simulink model "ex5_potentialFieldsTest_sim"  (R2025b)
settings: Solver=FixedStepAuto  StartTime=0.0  StopTime=15  FixedStep=1/GV.freq  RelTol=1e-3
values from neighbouring files (symbols this model uses):
  Kd = damp*w*2    (= 40)    [ex5_potentialFieldsTest.m]
  Kp = w*w    (= 400)    [ex5_potentialFieldsTest.m]
  vel_lim_max = 2.1750    (= 2.175)    [ex5_potentialFieldsTest.m]
  vel_lim_min = -vel_lim_max    (= -2.175)    [ex5_potentialFieldsTest.m]
libraries: simulink x1
settings Model: Creator=borek  LastModifiedBy=borek

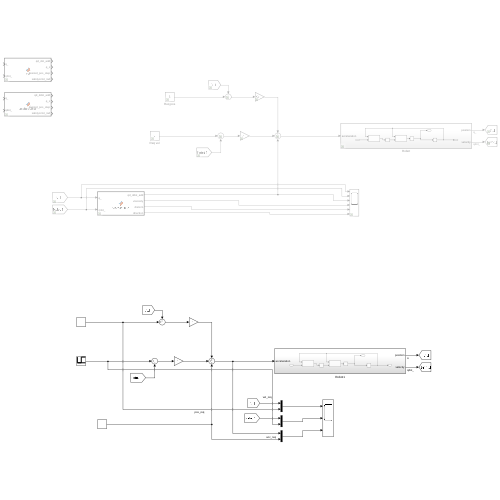
[thumbnail: Simulink's stored preview of the top-level diagram]
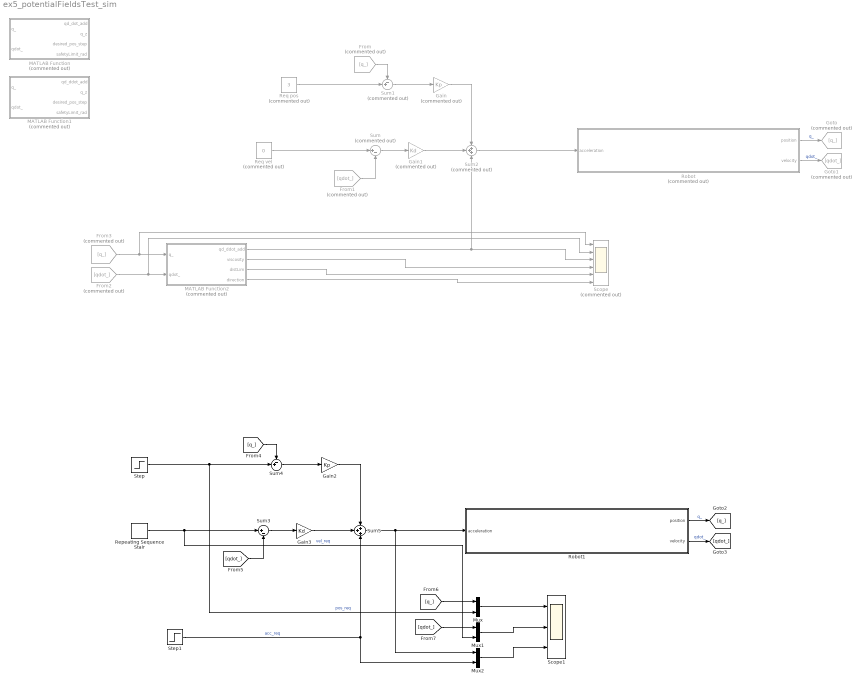
== system ex5_potentialFieldsTest_sim ==
  From : From  Commented=on  GotoTag=q_
  From1 : From  Commented=on  GotoTag=qdot_
  From2 : From  Commented=on  GotoTag=qdot_
  From3 : From  Commented=on  GotoTag=q_
  Gain : Gain  Commented=on  Gain=Kp
  Gain1 : Gain  Commented=on  Gain=Kd
  Gain2 : Gain  Gain=Kp
  Gain3 : Gain  Gain=Kd
  Goto : Goto  Commented=on  GotoTag=q_
  Goto1 : Goto  Commented=on  GotoTag=qdot_
  MATLAB Function : MATLAB Function  Commented=on  TreatAsAtomicUnit=on
  MATLAB Function1 : MATLAB Function  Commented=on  TreatAsAtomicUnit=on
  MATLAB Function2 : MATLAB Function  Commented=on  TreatAsAtomicUnit=on
  Mux : Mux  Inputs=2
  Mux1 : Mux  Inputs=2
  Mux2 : Mux  Inputs=2
  Repeating Sequence Stair : simulink/Sources/Repeating Sequence Stair  OutValues=[0 1].'  tsamp=4  OutMin=[]  OutMax=[]  OutDataTypeStr=double  OutputDataTypeScalingMode=double  OutDataType=fixdt(0,8)  ConRadixGroup=Best Precision: Vector-wise  OutScaling=2^-12
  Req pos : Constant  Commented=on  Value=3
  Req vel : Constant  Commented=on  Value=0
  Robot : Subsystem  Commented=on
  Robot1 : Subsystem
  Scope : Scope  Commented=on  NumInputPorts=6
      settings: ActiveDisplayYMinimum=-0.36189059089720149  ActiveDisplayYMaximum=3.257015318074814
  Scope1 : Scope  NumInputPorts=3
      settings: ActiveDisplayYMinimum=-0.20830211105695048  ActiveDisplayYMaximum=1.8747189995125548
  Step : Step  Time=6  SampleTime=0
  Step1 : Step  Time=10  After=-1*Kd  SampleTime=0
  Sum : Sum  Commented=on  Inputs=|+-
  Sum1 : Sum  Commented=on  Inputs=-+|
  Sum2 : Sum  Commented=on  Inputs=+++
  Sum3 : Sum  Inputs=|+-
  Sum4 : Sum  Inputs=-+|
  Sum5 : Sum  Inputs=+++
  wires:
  Req pos/1 -> Sum1/2
  Sum1/1 -> Gain/1
  Gain/1 -> Sum2/1
  Gain1/1 -> Sum2/2
  Sum/1 -> Gain1/1
  Sum2/1 -> Robot/1(acceleration)
  Req vel/1 -> Sum/1
  MATLAB Function2/1(qd_ddot_add) -> Scope/3, Sum2/3
  Robot/1(position) -> Goto/1  "q_"
  Robot/2(velocity) -> Goto1/1  "qdot_"
  From/1 -> Sum1/1
  From1/1 -> Sum/2
  From2/1 -> Scope/2, MATLAB Function2/2(qdot_)
  From3/1 -> Scope/1, MATLAB Function2/1(q_)
  MATLAB Function2/2(viscosity) -> Scope/4
  MATLAB Function2/3(distLim) -> Scope/5
  MATLAB Function2/4(direction) -> Scope/6
  Gain2/1 -> Sum5/1
  Sum3/1 -> Gain3/1
  Step1/1 -> Mux2/2, Sum5/3  "acc_req"
  Gain3/1 -> Sum5/2
  Step/1 -> Mux/2, Sum4/2  "pos_req"
  Sum5/1 -> Mux2/1, Robot1/1(acceleration)
  Repeating Sequence Stair/1 -> Mux1/2, Sum3/1  "vel_req"
  Robot1/1(position) -> [q_]  "q_"
  Robot1/2(velocity) -> [qdot_]  "qdot_"
  [q_] -> Sum4/1
  [qdot_] -> Sum3/2
  Sum4/1 -> Gain2/1
  Mux/1 -> Scope1/1
  Mux1/1 -> Scope1/2
  [q_] -> Mux/1
  [qdot_] -> Mux1/1
  Mux2/1 -> Scope1/3

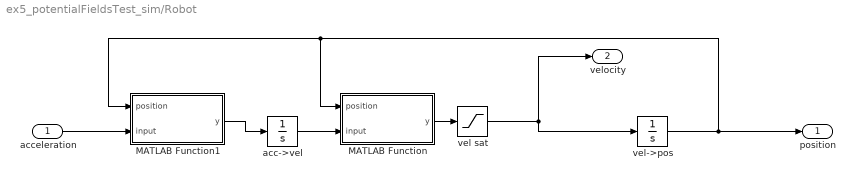
== system ex5_potentialFieldsTest_sim/Robot ==
  acceleration : Inport
  MATLAB Function : MATLAB Function  TreatAsAtomicUnit=on
  MATLAB Function1 : MATLAB Function  TreatAsAtomicUnit=on
  acc->vel : Integrator
  vel sat : Saturate  UpperLimit=vel_lim_max  LowerLimit=vel_lim_min
  vel->pos : Integrator
  position : Outport
  velocity : Outport  Port=2
  wires:
  vel->pos/1 -> MATLAB Function1/1(position), MATLAB Function/1(position), position/1
  vel sat/1 -> vel->pos/1, velocity/1
  acceleration/1 -> MATLAB Function1/2(input)
  acc->vel/1 -> MATLAB Function/2(input)
  MATLAB Function/1(y) -> vel sat/1
  MATLAB Function1/1(y) -> acc->vel/1

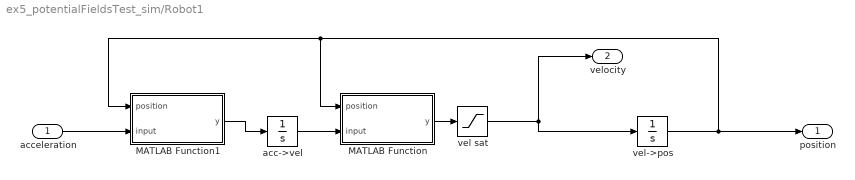
== system ex5_potentialFieldsTest_sim/Robot1 ==
  acceleration : Inport
  MATLAB Function : MATLAB Function  TreatAsAtomicUnit=on
  MATLAB Function1 : MATLAB Function  TreatAsAtomicUnit=on
  acc->vel : Integrator
  vel sat : Saturate  UpperLimit=vel_lim_max  LowerLimit=vel_lim_min
  vel->pos : Integrator
  position : Outport
  velocity : Outport  Port=2
  wires:
  vel->pos/1 -> MATLAB Function1/1(position), MATLAB Function/1(position), position/1
  vel sat/1 -> vel->pos/1, velocity/1
  acceleration/1 -> MATLAB Function1/2(input)
  acc->vel/1 -> MATLAB Function/2(input)
  MATLAB Function/1(y) -> vel sat/1
  MATLAB Function1/1(y) -> acc->vel/1

== matlab function ex5_potentialFieldsTest_sim/MATLAB Function1 ==
  data: q_ input; qd_ddot_add output; qdot_ input; GV parameter; q_z output; desired_pos_step output; safetyLimit_rad output
function [qd_ddot_add ,q_z,desired_pos_step,safetyLimit_rad] = accRepulsor(q_, qdot_, GV)

safetyLimit_deg = 10; % degrees
safetyLimit_rad = safetyLimit_deg * (3.14 / 180.0);% convert to radians
accelerationLimit = 10 ;%rad/s2
predictionCycles = 20;


disp("MaxSafetyLimit= " + num2str(-safetyLimit_rad+GV.pos_lim_max))

decayRate = 0.5; % decay rate
accCommandGain = 1; % velocity command gain

timeStep = predictionCycles/GV.freq

if qdot_ > 0 
    q_z  = q_  + (qdot_ * timeStep) - accelerationLimit*(timeStep*timeStep)*0.5
else
    q_z  = q_  + (qdot_ * timeStep) + accelerationLimit*(timeStep*timeStep)*0.5 
end

dist_max = (GV.pos_lim_max  - q_z )
dist_min = (GV.pos_lim_min  - q_z )

desired_pos_step = 0; % Initialize desired_pos_step
if (dist_max < safetyLimit_rad) && (qdot_  > 0)
desired_pos_step = (q_  - GV.pos_lim_max ) 
elseif (dist_min > -safetyLimit_rad) && (qdot_  < 0)
desired_pos_step = (q_  - GV.pos_lim_min )
end

qd_ddot_add  =  abs(desired_pos_step)*(desired_pos_step-qdot_*timeStep)/(timeStep*timeStep)*decayRate

== matlab function ex5_potentialFieldsTest_sim/MATLAB Function ==
  data: q_ input; qd_dot_add output; qdot_ input; GV parameter; q_z output; desired_pos_step output; safetyLimit_rad output
function [qd_dot_add ,q_z,desired_pos_step,safetyLimit_rad] = fcn(q_, qdot_, GV)

safetyLimit_deg = 10; % degrees
safetyLimit_rad = safetyLimit_deg * (3.14 / 180.0);% convert to radians
accelerationLimit = 10 ;%rad/s2
predictionCycles = 20;


disp("MaxSafetyLimit= " + num2str(-safetyLimit_rad+GV.pos_lim_max))

decayRate = 0.5; % decay rate
velCommandGain = 1; % velocity command gain

timeStep = predictionCycles/GV.freq

if qdot_ > 0 
    q_z  = q_  + (qdot_ * timeStep) - accelerationLimit*(timeStep*timeStep)*0.5
else
    q_z  = q_  + (qdot_ * timeStep) + accelerationLimit*(timeStep*timeStep)*0.5 
end

dist_max = (GV.pos_lim_max  - q_z )
dist_min = (GV.pos_lim_min  - q_z )

desired_pos_step = 0; % Initialize desired_pos_step
if (dist_max < safetyLimit_rad) && (qdot_  > 0)
desired_pos_step = (q_  - GV.pos_lim_max ) * decayRate
elseif (dist_min > -safetyLimit_rad) && (qdot_  < 0)
desired_pos_step = (q_  - GV.pos_lim_min ) * decayRate
end

qd_dot_add  = desired_pos_step * 1/timeStep * velCommandGain

== matlab function ex5_potentialFieldsTest_sim/MATLAB Function2 ==
  data: q_ input; qd_ddot_add output; qdot_ input; GV parameter; viscosity output; distLim output; direction output
function [qd_ddot_add ,viscosity,distLim,direction] = viscoseField(q_, qdot_, GV)

safetyLimit_deg = 10; % degrees
safetyLimit_rad = safetyLimit_deg * (3.14 / 180.0);% convert to radians
viscoseConstant = 50;







if qdot_ > 0
    direction = 1;
    distLim = q_-(GV.pos_lim_max-safetyLimit_rad);
elseif  qdot_ < 0
    direction = -1;
    distLim = q_-(GV.pos_lim_min+safetyLimit_rad);
else
    direction = 0;
    distLim = 0;
end

% distLim being positive means the field is active


if(distLim>0)
viscosity = (distLim*viscoseConstant)*(distLim*viscoseConstant);
else
viscosity = 0;
end

repulse = 0;
if(qdot_*direction > 0) % positive for heading in same direction = into the limit
    repulse = -qdot_ *  viscosity;
end


qd_ddot_add  =  repulse;

== matlab function ex5_potentialFieldsTest_sim/Robot/MATLAB Function ==
  data: position input; y output; input input; GV parameter
function y = posLimit(position, input, GV)



% GV.pos_lim_max = pos_lim_max;
% GV.pos_lim_min = pos_lim_min;

if position > GV.pos_lim_max
    
    if input > 0
        y = 0;
    else
        y= input;
    end

elseif position < GV.pos_lim_min
    
    if input < 0
        y = 0;
    else
        y= input;
    end

else
    y = input;

end

== matlab function ex5_potentialFieldsTest_sim/Robot/MATLAB Function1 ==
  data: position input; y output; input input; GV parameter
function y = posLimit(position, input, GV)



% GV.pos_lim_max = pos_lim_max;
% GV.pos_lim_min = pos_lim_min;

if position > GV.pos_lim_max
    
    if input > 0
        y = 0;
    else
        y= input;
    end

elseif position < GV.pos_lim_min
    
    if input < 0
        y = 0;
    else
        y= input;
    end

else
    y = input;

end

== matlab function ex5_potentialFieldsTest_sim/Robot1/MATLAB Function ==
  data: position input; y output; input input; GV parameter
function y = posLimit(position, input, GV)



% GV.pos_lim_max = pos_lim_max;
% GV.pos_lim_min = pos_lim_min;

if position > GV.pos_lim_max
    
    if input > 0
        y = 0;
    else
        y= input;
    end

elseif position < GV.pos_lim_min
    
    if input < 0
        y = 0;
    else
        y= input;
    end

else
    y = input;

end

== matlab function ex5_potentialFieldsTest_sim/Robot1/MATLAB Function1 ==
  data: position input; y output; input input; GV parameter
function y = posLimit(position, input, GV)



% GV.pos_lim_max = pos_lim_max;
% GV.pos_lim_min = pos_lim_min;

if position > GV.pos_lim_max
    
    if input > 0
        y = 0;
    else
        y= input;
    end

elseif position < GV.pos_lim_min
    
    if input < 0
        y = 0;
    else
        y= input;
    end

else
    y = input;

end
